simulink model "Encoder_Block_Diagram"  (R2016b)
settings: Solver=VariableStepAuto  StartTime=0.0  StopTime=10.0  RelTol=1e-3
settings Model: Creator=silviobacci  LastModifiedBy=silviobacci

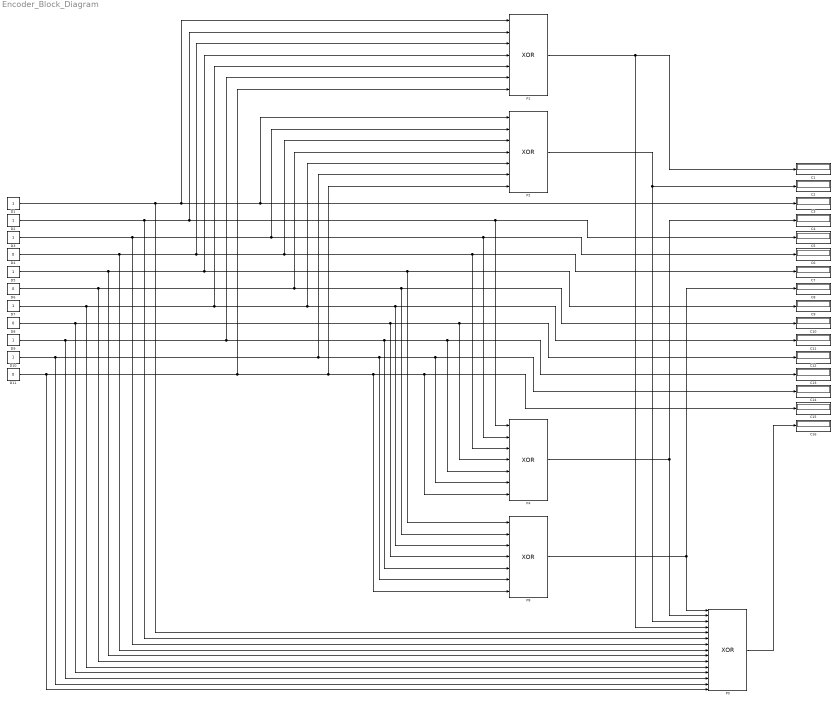
== system Encoder_Block_Diagram ==
  C{1..16} (16 alike) : Display
  D{1..3,5,7,9..10} (7 alike) : Constant  OutDataTypeStr=boolean
  D{4,6,8,11} (4 alike) : Constant  Value=0  OutDataTypeStr=boolean
  P0 : Logic  Operator=XOR  Inputs=15  AllPortsSameDT=off  OutDataTypeStr=boolean
  P{1..2,4,8} (4 alike) : Logic  Operator=XOR  Inputs=7  AllPortsSameDT=off  OutDataTypeStr=boolean
  wires:
  D3/1 -> P0/7, P2/2, C6/1, P4/2
  P1/1 -> C1/1, P0/4
  P2/1 -> P0/3, C2/1
  P4/1 -> P0/2, C4/1
  P8/1 -> P0/1, C8/1
  D1/1 -> P0/5, P1/1, C3/1, P2/1
  D2/1 -> P0/6, P1/2, C5/1, P4/1
  D4/1 -> P0/8, P1/3, P2/3, C7/1, P4/3
  D5/1 -> P0/9, P1/4, C9/1, P8/1
  D6/1 -> P0/10, P2/4, C10/1, P8/2
  D7/1 -> P0/11, P1/5, P2/5, C11/1, P8/3
  D8/1 -> P0/12, P8/4, C12/1, P4/4
  D9/1 -> P0/13, P1/6, P8/5, C13/1, P4/5
  D10/1 -> P0/14, P2/6, P8/6, C14/1, P4/6
  D11/1 -> P0/15, P1/7, P2/7, P8/7, C15/1, P4/7
  P0/1 -> C16/1
